simulink model "LinearVNonLinear"  (R2024a)
settings: Solver=VariableStepAuto  StartTime=0.0  StopTime=10.0  RelTol=1e-3
undefined symbols (not defined in the file or in its folder): Lamda, Ld, Lq, Rs
settings Model: Creator=nicco  LastModifiedBy=nicco

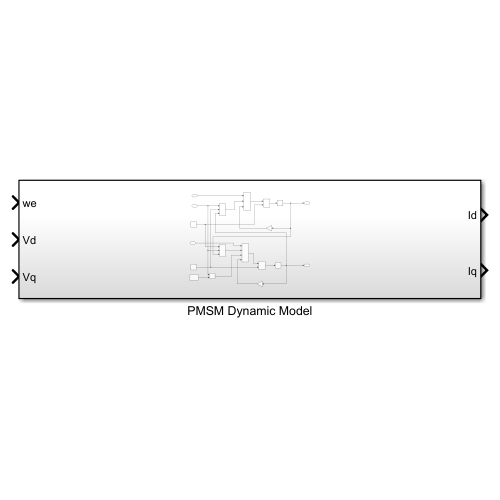
[thumbnail: Simulink's stored preview of the top-level diagram]
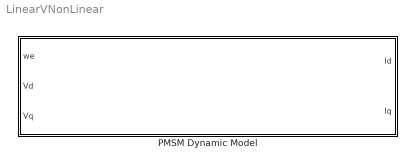
== system LinearVNonLinear ==
  PMSM Dynamic Model : Subsystem

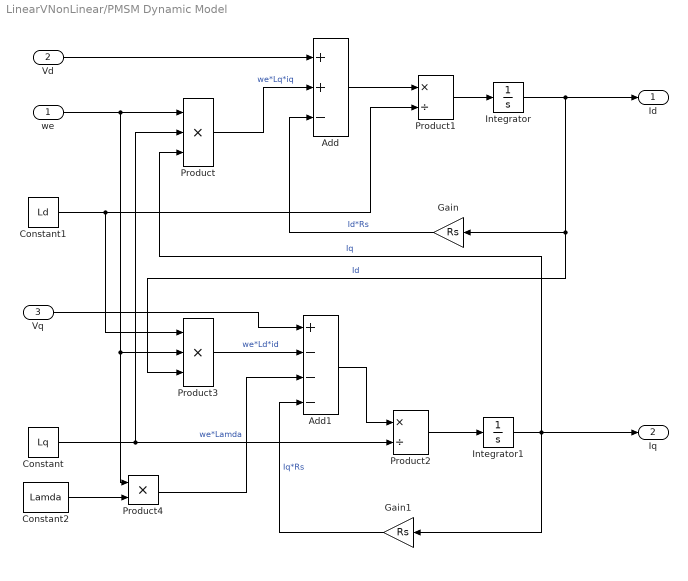
== system LinearVNonLinear/PMSM Dynamic Model ==
  we : Inport
  Vd : Inport  Port=2
  Vq : Inport  Port=3
  Add : Sum  Inputs=++-
  Add1 : Sum  Inputs=+---
  Constant : Constant  Value=Lq
  Constant1 : Constant  Value=Ld
  Constant2 : Constant  Value=Lamda
  Gain : Gain  Gain=Rs
  Gain1 : Gain  Gain=Rs
  Integrator : Integrator
  Integrator1 : Integrator
  Product : Product  Inputs=3
  Product1 : Product  Inputs=*/
  Product2 : Product  Inputs=*/
  Product3 : Product  Inputs=3
  Product4 : Product  Inputs=**
  Id : Outport
  Iq : Outport  Port=2
  wires:
  Vd/1 -> Add/1
  Integrator/1 -> Id/1, Product3/3, Gain/1  "Id"
  Integrator1/1 -> Iq/1, Gain1/1, Product/3  "Iq"
  Constant/1 -> Product/2, Product2/2
  we/1 -> Product4/1, Product3/2, Product/1
  Constant2/1 -> Product4/2
  Constant1/1 -> Product3/1, Product1/2
  Product2/1 -> Integrator1/1
  Vq/1 -> Add1/1
  Gain1/1 -> Add1/4  "Iq*Rs"
  Product4/1 -> Add1/3  "we*Lamda"
  Add/1 -> Product1/1
  Product1/1 -> Integrator/1
  Gain/1 -> Add/3  "Id*Rs"
  Add1/1 -> Product2/1
  Product/1 -> Add/2  "we*Lq*iq"
  Product3/1 -> Add1/2  "we*Ld*id"
